simulink model "Diagrama_invernadero_tradicional"  (R2019b)
settings: Solver=VariableStepAuto  StartTime=0.0  StopTime=24  RelTol=1e-3
libraries: Libreria x10
settings Model: Creator=Usuario  LastModifiedBy=PC-01
settings SFSimCC: CustomCodeUndefinedFunction=UseInterfaceOnly

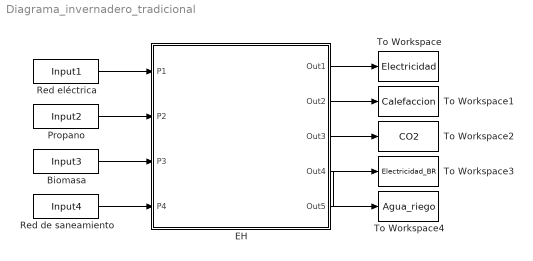
== system Diagrama_invernadero_tradicional ==
  Biomasa : FromWorkspace  VariableName=Input3  SampleTime=0
  EH : Subsystem
  Propano : FromWorkspace  VariableName=Input2  SampleTime=0
  Red de saneamiento : FromWorkspace  VariableName=Input4  SampleTime=0
  Red eléctrica : FromWorkspace  VariableName=Input1  SampleTime=0
  To Workspace : ToWorkspace  VariableName=Electricidad  SaveFormat=Timeseries  SampleTime=-1
  To Workspace1 : ToWorkspace  VariableName=Calefaccion  SaveFormat=Timeseries  SampleTime=-1
  To Workspace2 : ToWorkspace  VariableName=CO2  SaveFormat=Timeseries  SampleTime=-1
  To Workspace3 : ToWorkspace  VariableName=Electricidad_BR  SaveFormat=Timeseries  SampleTime=-1
  To Workspace4 : ToWorkspace  VariableName=Agua_riego  SaveFormat=Timeseries  SampleTime=-1
  wires:
  Red eléctrica/1 -> EH/1(P1)
  Propano/1 -> EH/2(P2)
  Biomasa/1 -> EH/3(P3)
  Red de saneamiento/1 -> EH/4(P4)
  EH/1(Out1) -> To Workspace/1
  EH/2(Out2) -> To Workspace1/1
  EH/3(Out3) -> To Workspace2/1
  EH/5(Out5) -> To Workspace3/1
  EH/4(Out4) -> To Workspace4/1

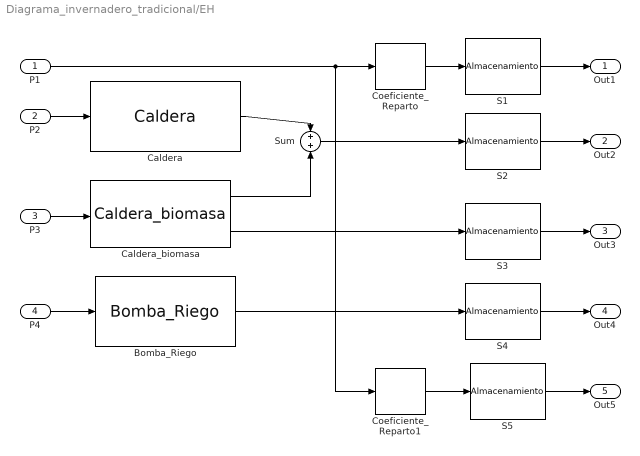
== system Diagrama_invernadero_tradicional/EH ==
  P1 : Inport
  P2 : Inport  Port=2
  P3 : Inport  Port=3
  P4 : Inport  Port=4
  Bomba_Riego : Libreria/Bomba_Riego  efficiency=1  dispatch_factor=beta1  T_muestreo=T_muestreo  Max_in=150  Max_out=150  n_salida=[5]
      link override Funcion_coef_reparto: Tm=T_muestreo
  Caldera : Libreria/Caldera  efficiency=11.54  dispatch_factor=1  T_muestreo=T_muestreo  Min_in=0  Max_in=6.8  Max_out=78.472
  Caldera_biomasa : Libreria/Caldera_biomasa  efficiency=[4.25 1.76]  dispatch_factor=1  T_muestreo=T_muestreo  Max_in=40  Min_in=1  Max_out=[170 70.4]
  Coeficiente_Reparto : Libreria/Coeficiente_Reparto  dispatch_factor=alfa1  Tm=T_muestreo  Max_out=inf  Max_in=inf  efficiency=1
  Coeficiente_Reparto1 : Libreria/Coeficiente_Reparto  dispatch_factor=alfa2  Tm=T_muestreo  Max_out=inf  Max_in=inf  efficiency=1
  S1 : Libreria/Almacenamiento  Up2=1000  Low2=0  r_c=1  Up=1000  Low=0  r_d=1  Up1=1000  Low1=0  almacenamiento_inicial=0  cpa=0  almacenamiento_on=on
      link override In1: SampleTime=1
      link override Qch: VariableName=Qchp1
      link override Qdis: VariableName=Qdisp1
      link override almacenamiento: VariableName=almacen1
      link override discrepancias_almacenamiento: VariableName=discrepancias_almacenamiento1
      link override ef: VariableName=Ech1
      link override eff: VariableName=Edis1
  S2 : Libreria/Almacenamiento  Up2=104.5  Low2=0  r_c=0.9  Up=104.5  Low=0  r_d=0.9  Up1=174.2  Low1=0  almacenamiento_inicial=0  cpa=0.06  almacenamiento_on=on
      link override In1: SampleTime=1
      link override Qch: VariableName=Qchp2
      link override Qdis: VariableName=Qdisp2
      link override almacenamiento: VariableName=almacen2
      link override discrepancias_almacenamiento: VariableName=discrepancias_almacenamiento2
      link override ef: VariableName=Ech2
      link override eff: VariableName=Edis2
  S3 : Libreria/Almacenamiento  Up2=51  Low2=0  r_c=1  Up=51  Low=0  r_d=1  Up1=25.2  Low1=0  almacenamiento_inicial=0  cpa=0  almacenamiento_on=on
      link override In1: SampleTime=1
      link override Qch: VariableName=Qchp3
      link override Qdis: VariableName=Qdisp3
      link override almacenamiento: VariableName=almacen3
      link override discrepancias_almacenamiento: VariableName=discrepancias_almacenamiento3
      link override ef: VariableName=Ech3
      link override eff: VariableName=Edis3
  S4 : Libreria/Almacenamiento  Up2=100  Low2=0  r_c=1  Up=250  Low=0  r_d=1  Up1=1000  Low1=0  almacenamiento_inicial=0  cpa=0  almacenamiento_on=on
      link override In1: SampleTime=1
      link override Qch: VariableName=Qchp4
      link override Qdis: VariableName=Qdisp4
      link override almacenamiento: VariableName=almacen5
      link override discrepancias_almacenamiento: VariableName=discrepancias_almacenamiento5
      link override ef: VariableName=Ech4
      link override eff: VariableName=Edis4
  S5 : Libreria/Almacenamiento  Up2=1000  Low2=0  r_c=1  Up=1000  Low=0  r_d=1  Up1=1000  Low1=0  almacenamiento_inicial=0  cpa=0  almacenamiento_on=on
      link override In1: SampleTime=1
      link override Qch: VariableName=Qchp5
      link override Qdis: VariableName=Qdisp5
      link override almacenamiento: VariableName=almacen4
      link override discrepancias_almacenamiento: VariableName=discrepancias_almacenamiento4
      link override ef: VariableName=Ech5
      link override eff: VariableName=Edis5
  Sum : Sum
  Out1 : Outport  VectorParamsAs1DForOutWhenUnconnected=off
  Out2 : Outport  Port=2  VectorParamsAs1DForOutWhenUnconnected=off
  Out3 : Outport  Port=3  VectorParamsAs1DForOutWhenUnconnected=off
  Out4 : Outport  Port=4  VectorParamsAs1DForOutWhenUnconnected=off
  Out5 : Outport  Port=5  VectorParamsAs1DForOutWhenUnconnected=off
  wires:
  Caldera/1 -> Sum/1
  Coeficiente_Reparto/1 -> S1/1
  Coeficiente_Reparto1/1 -> S5/1
  Bomba_Riego/1 -> S4/1
  Sum/1 -> S2/1
  S4/1 -> Out4/1
  P1/1 -> Coeficiente_Reparto1/1, Coeficiente_Reparto/1
  Caldera_biomasa/2 -> S3/1
  Caldera_biomasa/1 -> Sum/2
  S5/1 -> Out5/1
  S3/1 -> Out3/1
  P4/1 -> Bomba_Riego/1
  P3/1 -> Caldera_biomasa/1
  P2/1 -> Caldera/1
  S2/1 -> Out2/1
  S1/1 -> Out1/1
